simulink model "TLC_model"  (R2019a)
settings: Solver=FixedStepDiscrete  StartTime=0.0  StopTime=40  FixedStep=0.25  RelTol=1e-3
undefined symbols (not defined in the file): sigbuilder_block
settings Model: EnablePacing=on  PacingRate=3  Creator=Athar Hussain  LastModifiedBy=Athar Hussain

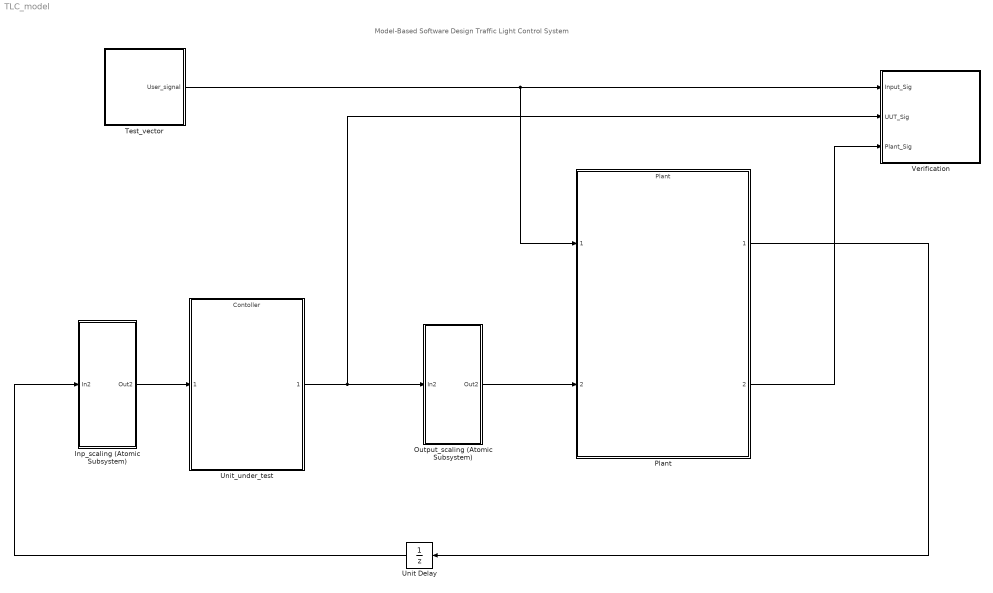
== system TLC_model ==
  note: Model-Based Software Design
      | Traffic Light Control System
  Inp_scaling (Atomic Subsystem) : Subsystem  TreatAsAtomicUnit=on
  Output_scaling (Atomic Subsystem) : Subsystem  TreatAsAtomicUnit=on
  Plant : ModelReference  ModelNameDialog=Plant.slx  SimulationMode=Normal  ModelReferenceVersion=1.40
  "Test_vector " : Subsystem
  Unit Delay : UnitDelay  SampleTime=-1  HasFrameUpgradeWarning=on
  Unit_under_test : ModelReference  ModelNameDialog=Contoller.slx  SimulationMode=Normal  ModelReferenceVersion=1.80
  Verification : Subsystem
  wires:
  Unit_under_test/1 -> Verification/2(UUT_Sig), Output_scaling (Atomic Subsystem)/1(In2)
  Plant/1 -> Unit Delay/1
  Output_scaling (Atomic Subsystem)/1(Out2) -> Plant/2
  Plant/2 -> Verification/3(Plant_Sig)
  Inp_scaling (Atomic Subsystem)/1(Out2) -> Unit_under_test/1
  Unit Delay/1 -> Inp_scaling (Atomic Subsystem)/1(In2)
  "Test_vector "/1(User_signal) -> Plant/1, Verification/1(Input_Sig)

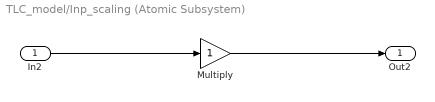
== system TLC_model/Inp_scaling (Atomic Subsystem) ==
  In2 : Inport
  Multiply : Gain
  Out2 : Outport
  wires:
  Multiply/1 -> Out2/1
  In2/1 -> Multiply/1

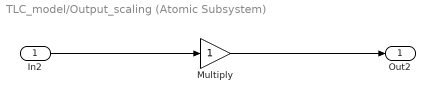
== system TLC_model/Output_scaling (Atomic Subsystem) ==
  In2 : Inport
  Multiply : Gain
  Out2 : Outport
  wires:
  Multiply/1 -> Out2/1
  In2/1 -> Multiply/1

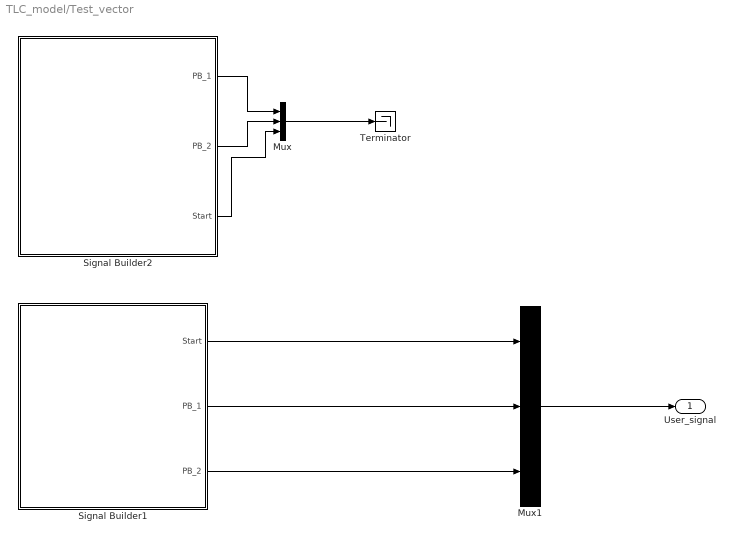
== system TLC_model/Test_vector  ==
  Mux : Mux  Inputs=3
  Mux1 : Mux  Inputs=3
  Signal Builder1 : Subsystem  Tag=STV Subsys  LoadFcn=sigbuilder_block('load');  StartFcn=sigbuilder_block('start');  StopFcn=sigbuilder_block('stop');  ClipboardFcn=sigbuilder_block('clipboard');  mask(Sigbuilder block){tuvar=[0:10]}
      mask help: Simulink:masks:SigbuilderBlock_MD
      mask init:
      | if ~strcmp(get_param(bdroot(gcbh),'SimulationStatus'),'stopped') tuvar = sigbuilder_block('maskInit'); end
      settings: CopyFcn=sigbuilder_block('copy');  DeleteFcn=sigbuilder_block('delete');  ModelCloseFcn=sigbuilder_block('modelClose');  PreSaveFcn=sigbuilder_block('preSave');  PauseFcn=sigbuilder_block('pause');  ContinueFcn=sigbuilder_block('continue');  NameChangeFcn=sigbuilder_block('namechange');  OpenFcn=sigbuilder_block('open',[5.4 51.6 1141.2 490.8 ]);  CloseFcn=sigbuilder_block('close');
      mask Display: plot(0, 0, 100, 100,[2, 2, 32, 32, 2], [68, 8, 8, 68, 68],[32, 2], [38, 38], [32, 19, 2],[53, 60, 44], [32, 17, 17, 2],[16, 16, 31, 31]);txt = getActiveGroup(gcbh);text(2, 100, txt,'verticalAlignment', 'top');
  Signal Builder2 : Subsystem  Tag=STV Subsys  LoadFcn=sigbuilder_block('load');  StartFcn=sigbuilder_block('start');  StopFcn=sigbuilder_block('stop');  ClipboardFcn=sigbuilder_block('clipboard');  mask(Sigbuilder block){tuvar=[0:10]}
      mask help: Simulink:masks:SigbuilderBlock_MD
      mask init:
      | if ~strcmp(get_param(bdroot(gcbh),'SimulationStatus'),'stopped') tuvar = sigbuilder_block('maskInit'); end
      settings: CopyFcn=sigbuilder_block('copy');  DeleteFcn=sigbuilder_block('delete');  ModelCloseFcn=sigbuilder_block('modelClose');  PreSaveFcn=sigbuilder_block('preSave');  PauseFcn=sigbuilder_block('pause');  ContinueFcn=sigbuilder_block('continue');  NameChangeFcn=sigbuilder_block('namechange');  OpenFcn=sigbuilder_block('open',[5.4 9 1141.2 451.8 ]);  CloseFcn=sigbuilder_block('close');
      mask Display: plot(0, 0, 100, 100,[2, 2, 32, 32, 2], [68, 8, 8, 68, 68],[32, 2], [38, 38], [32, 19, 2],[53, 60, 44], [32, 17, 17, 2],[16, 16, 31, 31]);txt = getActiveGroup(gcbh);text(2, 100, txt,'verticalAlignment', 'top');
  Terminator : Terminator
  User_signal : Outport
  wires:
  Signal Builder1/3(PB_2) -> Mux1/3
  Signal Builder1/2(PB_1) -> Mux1/2
  Signal Builder1/1(Start) -> Mux1/1
  Mux1/1 -> User_signal/1
  Signal Builder2/1(PB_1) -> Mux/1
  Signal Builder2/2(PB_2) -> Mux/2
  Signal Builder2/3(Start) -> Mux/3
  Mux/1 -> Terminator/1

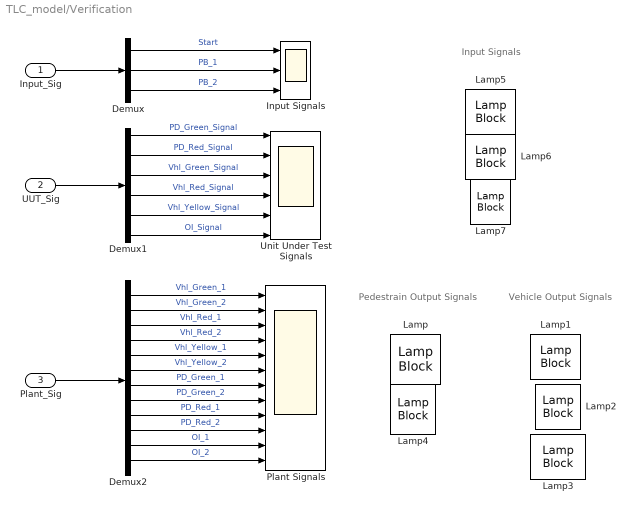
== system TLC_model/Verification ==
  note: Vehicle Output Signals
  note: Pedestrain Output Signals
  note: Input Signals
  Input_Sig : Inport
  UUT_Sig : Inport  Port=2
  Plant_Sig : Inport  Port=3
  Demux : Demux  Outputs=3
  Demux1 : Demux  Outputs=6
  Demux2 : Demux  Outputs=12
  Input Signals : Scope  NumInputPorts=3
  Lamp{,1..7} (8 alike) : LampBlock
  Plant Signals : Scope  NumInputPorts=12
  Unit Under Test Signals : Scope  NumInputPorts=6
  wires:
  Input_Sig/1 -> Demux/1
  Demux1/1 -> Unit Under Test Signals/1  "PD_Green_Signal"
  Demux1/2 -> Unit Under Test Signals/2  "PD_Red_Signal"
  Demux1/3 -> Unit Under Test Signals/3  "Vhl_Green_Signal"
  Demux1/4 -> Unit Under Test Signals/4  "Vhl_Red_Signal"
  Demux1/5 -> Unit Under Test Signals/5  "Vhl_Yellow_Signal"
  Demux1/6 -> Unit Under Test Signals/6  "OI_Signal"
  UUT_Sig/1 -> Demux1/1
  Demux2/1 -> Plant Signals/1  "Vhl_Green_1"
  Demux2/2 -> Plant Signals/2  "Vhl_Green_2"
  Demux2/3 -> Plant Signals/3  "Vhl_Red_1"
  Demux2/4 -> Plant Signals/4  "Vhl_Red_2"
  Demux2/5 -> Plant Signals/5  "Vhl_Yellow_1"
  Demux2/6 -> Plant Signals/6  "Vhl_Yellow_2"
  Demux2/7 -> Plant Signals/7  "PD_Green_1"
  Demux2/8 -> Plant Signals/8  "PD_Green_2"
  Demux2/9 -> Plant Signals/9  "PD_Red_1"
  Demux2/10 -> Plant Signals/10  "PD_Red_2"
  Demux2/11 -> Plant Signals/11  "OI_1"
  Demux2/12 -> Plant Signals/12  "OI_2"
  Plant_Sig/1 -> Demux2/1
  Demux/1 -> Input Signals/1  "Start"
  Demux/2 -> Input Signals/2  "PB_1"
  Demux/3 -> Input Signals/3  "PB_2"

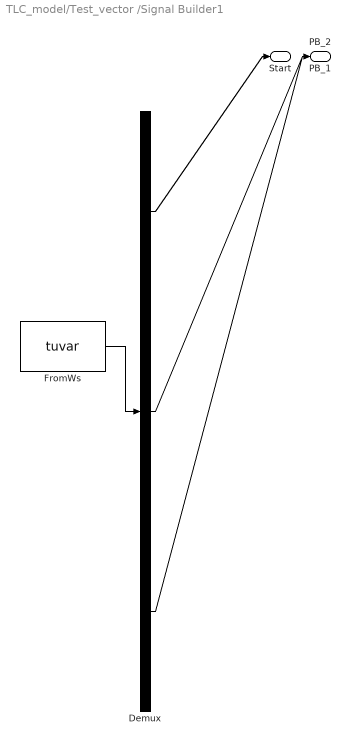
== system TLC_model/Test_vector /Signal Builder1 ==
  Demux : Demux  Tag=STV Demux  Outputs=3
  FromWs : FromWorkspace  Tag=STV FromWs  VariableName=tuvar  SampleTime=0
      SigBuilderData=|
      | common.afterFinalStr = 'Extrapolate'
      | common.sampleTime = 0
      | dataSet(1).timeRange = [0 42]
      | dataSet(1).name = 'Test_case_1'
      | dataSet(2).timeRange = [0 42]
      | dataSet(2).name = 'Test_case_2'
      | dataSet(3).timeRange = [0 42]
      | dataSet(3).name = 'Test_case_3'
      | dataSet(4).timeRange = [0 42]
      | dataSet(4).name = 'Test_case_4'
      | dataSet(5).timeRange = [0 42]
      | dataSet(5).name = 'Test_case_5'
      | sbobj.Groups(1).Name = 'Test_case_1'
      | sbobj.Groups(1).Signals(1).Name = 'Start'
      | sbobj.Groups(1).Signals(1).XData = [0 1.75 1.75 42]
      | sbobj.Groups(1).Signals(1).YData = [0 0 1 1]
      | sbobj.Groups(1).Signals(2).Name = 'PB_1'
      | sbobj.Groups(1).Signals(2).XData = [0 14 14 15 15 42]
      | sbobj.Groups(1).Signals(2).YData = [0 0 1 1 0 0]
      | sbobj.Groups(1).Signals(3).Name = 'PB_2'
      | sbobj.Groups(1).Signals(3).XData = [0 16 16 17 17 42]
      | sbobj.Groups(1).Signals(3).YData = [0 0 1 1 0 0]
      | sbobj.Groups(1).TimeRange = [0 42]
      | sbobj.Groups(2).Name = 'Test_case_2'
      | sbobj.Groups(2).Signals(1).Name = 'Start'
      | sbobj.Groups(2).Signals(1).XData = [0 1.75 1.75 42]
      | sbobj.Groups(2).Signals(1).YData = [0 0 1 1]
      | sbobj.Groups(2).Signals(2).Name = 'PB_1'
      | sbobj.Groups(2).Signals(2).XData = [0 14 14 15 15 42]
      | sbobj.Groups(2).Signals(2).YData = [0 0 1 1 0 0]
      | sbobj.Groups(2).Signals(3).Name = 'PB_2'
      | sbobj.Groups(2).Signals(3).XData = [0 14 14 15 15 42]
      | sbobj.Groups(2).Signals(3).YData = [0 0 1 1 0 0]
      | sbobj.Groups(2).TimeRange = [0 42]
      | sbobj.Groups(3).Name = 'Test_case_3'
      | sbobj.Groups(3).Signals(1).Name = 'Start'
      | sbobj.Groups(3).Signals(1).XData = [0 1.75 1.75 42]
      | sbobj.Groups(3).Signals(1).YData = [0 0 1 1]
      | sbobj.Groups(3).Signals(2).Name = 'PB_1'
      | sbobj.Groups(3).Signals(2).XData = [0 14 14 15 15 42]
      | sbobj.Groups(3).Signals(2).YData = [0 0 1 1 0 0]
      | sbobj.Groups(3).Signals(3).Name = 'PB_2'
      | sbobj.Groups(3).Signals(3).XData = [0 42]
      | sbobj.Groups(3).Signals(3).YData = [0 0]
      | sbobj.Groups(3).TimeRange = [0 42]
      | sbobj.Groups(4).Name = 'Test_case_4'
      | sbobj.Groups(4).Signals(1).Name = 'Start'
      | sbobj.Groups(4).Signals(1).XData = [0 1.75 1.75 42]
      | sbobj.Groups(4).Signals(1).YData = [0 0 1 1]
      | sbobj.Groups(4).Signals(2).Name = 'PB_1'
      | sbobj.Groups(4).Signals(2).XData = [0 42]
      | sbobj.Groups(4).Signals(2).YData = [0 0]
      | sbobj.Groups(4).Signals(3).Name = 'PB_2'
      | sbobj.Groups(4).Signals(3).XData = [0 14 14 15 15 42]
      | sbobj.Groups(4).Signals(3).YData = [0 0 1 1 0 0]
      | sbobj.Groups(4).TimeRange = [0 42]
      | sbobj.Groups(5).Name = 'Test_case_5'
      | sbobj.Groups(5).Signals(1).Name = 'Start'
      | sbobj.Groups(5).Signals(1).XData = [0 1.75 1.75 42]
      | sbobj.Groups(5).Signals(1).YData = [0 0 1 1]
      | sbobj.Groups(5).Signals(2).Name = 'PB_1'
      | sbobj.Groups(5).Signals(2).XData = [0 25 26 42]
      | sbobj.Groups(5).Signals(2).YData = [0 0 0 0]
      | sbobj.Groups(5).Signals(3).Name = 'PB_2'
      | sbobj.Groups(5).Signals(3).XData = [0 40 42]
      | sbobj.Groups(5).Signals(3).YData = [0 0 0]
      | sbobj.Groups(5).TimeRange = [0 42]
  Start : Outport  Tag=STV Outport
  PB_1 : Outport  Tag=STV Outport  Port=2
  PB_2 : Outport  Tag=STV Outport  Port=3
  wires:
  FromWs/1 -> Demux/1
  Demux/1 -> Start/1
  Demux/2 -> PB_1/1
  Demux/3 -> PB_2/1

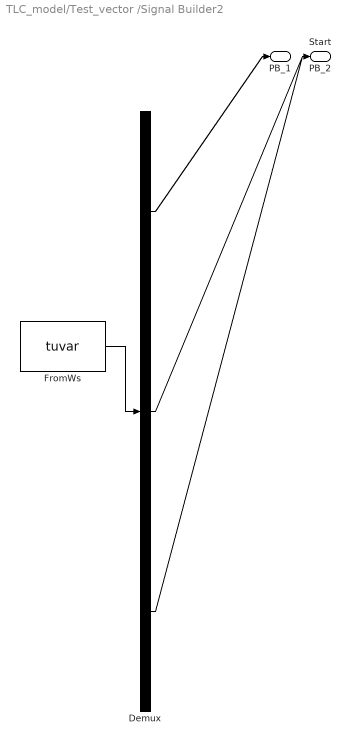
== system TLC_model/Test_vector /Signal Builder2 ==
  Demux : Demux  Tag=STV Demux  Outputs=3
  FromWs : FromWorkspace  Tag=STV FromWs  VariableName=tuvar  SampleTime=0
      SigBuilderData=|
      | common.afterFinalStr = 'Extrapolate'
      | common.sampleTime = 0
      | dataSet(1).timeRange = [0 42]
      | dataSet(1).name = 'Test_case_6'
      | dataSet(2).timeRange = [0 42]
      | dataSet(2).name = 'Test_case_7'
      | sbobj.Groups(1).Name = 'Test_case_6'
      | sbobj.Groups(1).Signals(1).Name = 'PB_1'
      | sbobj.Groups(1).Signals(1).XData = [0 2 4 6 8 10 12 15 15 16 16 18 20 22 24 24 25 25 30 32 34 36 38 40 42]
      | sbobj.Groups(1).Signals(1).YData = [0 0 0 0 0 0 0 0 1 1 0 0 0 0 0 1 1 0 0 0 0 0 0 0 0]
      | sbobj.Groups(1).Signals(2).Name = 'PB_2'
      | sbobj.Groups(1).Signals(2).XData = [0 2 4 6 8 10 12 14 16 18 18 19 19 24 27 27 28 28 32 34 36 38 40 42]
      | sbobj.Groups(1).Signals(2).YData = [0 0 0 0 0 0 0 0 0 0 1 1 0 0 0 1 1 0 0 0 0 0 0 0]
      | sbobj.Groups(1).Signals(3).Name = 'Start'
      | sbobj.Groups(1).Signals(3).XData = [0 1.75 1.75 4 6 8 12 14 16 18 20 22 24 26 28 30 32 34 36 38 40 42]
      | sbobj.Groups(1).Signals(3).YData = [0 0 1 1 1 1 1 1 1 1 1 1 1 1 1 1 1 1 1 1 1 1]
      | sbobj.Groups(1).TimeRange = [0 42]
      | sbobj.Groups(2).Name = 'Test_case_7'
      | sbobj.Groups(2).Signals(1).Name = 'PB_1'
      | sbobj.Groups(2).Signals(1).XData = [0 2 4 6 8 10 12 15 16 18 20 22 24 25 30 32 34 36 38 40 42]
      | sbobj.Groups(2).Signals(1).YData = [0 0 0 0 0 0 0 0 0 0 0 0 0 0 0 0 0 0 0 0 0]
      | sbobj.Groups(2).Signals(2).Name = 'PB_2'
      | sbobj.Groups(2).Signals(2).XData = [0 2 4 6 8 10 12 14 16 18 19 24 27 28 32 34 36 38 40 42]
      | sbobj.Groups(2).Signals(2).YData = [0 0 0 0 0 0 0 0 0 0 0 0 0 0 0 0 0 0 0 0]
      | sbobj.Groups(2).Signals(3).Name = 'Start'
      | sbobj.Groups(2).Signals(3).XData = [0 2 4 6 8 10 12 14 16 18 20 22 24 26 28 30 32 34 36 38 40 42]
      | sbobj.Groups(2).Signals(3).YData = [0 0 0 0 0 0 0 0 0 0 0 0 0 0 0 0 0 0 0 0 0 0]
      | sbobj.Groups(2).TimeRange = [0 42]
  PB_1 : Outport  Tag=STV Outport
  PB_2 : Outport  Tag=STV Outport  Port=2
  Start : Outport  Tag=STV Outport  Port=3
  wires:
  FromWs/1 -> Demux/1
  Demux/1 -> PB_1/1
  Demux/2 -> PB_2/1
  Demux/3 -> Start/1
